simulink model "test_stepper"  (R2020b)
settings: Solver=VariableStepAuto  StartTime=0.0  StopTime=10.0  RelTol=1e-3
undefined symbols (not defined in the file): stepper
settings Model: Creator=Utente  LastModifiedBy=Utente
settings SolverCC: ZeroCrossAlgorithm=Adaptive
settings DebuggingCC: IgnoredZcDiagnostic=none

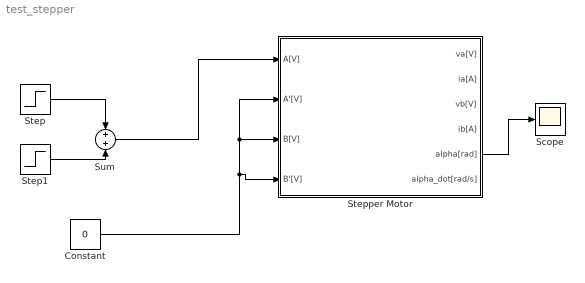
== system test_stepper ==
  Constant : Constant  Value=0
  Scope : Scope
  Step : Step  Time=0  After=9  SampleTime=0
  Step1 : Step  Time=0.0001  After=-1  SampleTime=0
  Stepper Motor : Subsystem
  Sum : Sum
  wires:
  Step/1 -> Sum/1
  Step1/1 -> Sum/2
  Sum/1 -> Stepper Motor/1(A[V])
  Constant/1 -> Stepper Motor/4(B'[V]), Stepper Motor/3(B[V]), Stepper Motor/2(A'[V])
  Stepper Motor/5(alpha[rad]) -> Scope/1

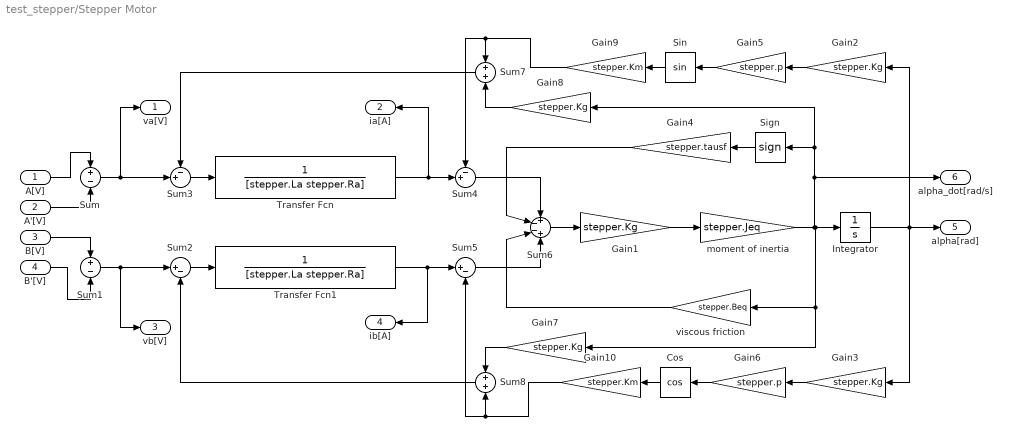
== system test_stepper/Stepper Motor ==
  A[V] : Inport
  A'[V] : Inport  Port=2
  B[V] : Inport  Port=3
  B'[V] : Inport  Port=4
  Cos : Trigonometry  Operator=cos
  Gain{1..3,7..8} (5 alike) : Gain  Gain=stepper.Kg
  Gain10 : Gain  Gain=stepper.Km
  Gain4 : Gain  Gain=stepper.tausf
  Gain5 : Gain  Gain=stepper.p
  Gain6 : Gain  Gain=stepper.p
  Gain9 : Gain  Gain=stepper.Km
  Integrator : Integrator
  Sign : Signum  ZeroCross=off
  Sin : Trigonometry
  Sum : Sum  Inputs=+|-
  Sum1 : Sum  Inputs=+|-
  Sum2 : Sum  Inputs=|+-
  Sum3 : Sum  Inputs=-+|
  Sum4 : Sum  Inputs=-+|
  Sum5 : Sum  Inputs=|+-
  Sum6 : Sum  Inputs=+--+
  Sum7 : Sum
  Sum8 : Sum
  Transfer Fcn : TransferFcn  Denominator=[stepper.La stepper.Ra]
  Transfer Fcn1 : TransferFcn  Denominator=[stepper.La stepper.Ra]
  moment of inertia : Gain  Gain=stepper.Jeq
  viscous friction : Gain  Gain=stepper.Beq
  va[V] : Outport
  ia[A] : Outport  Port=2
  vb[V] : Outport  Port=3
  ib[A] : Outport  Port=4
  alpha[rad] : Outport  Port=5
  alpha_dot[rad/s] : Outport  Port=6
  wires:
  A'[V]/1 -> Sum/2
  A[V]/1 -> Sum/1
  Sum/1 -> Sum3/2, va[V]/1
  B[V]/1 -> Sum1/1
  B'[V]/1 -> Sum1/2
  Sum1/1 -> Sum2/1, vb[V]/1
  Integrator/1 -> Gain3/1, Gain2/1, alpha[rad]/1
  Sum3/1 -> Transfer Fcn/1
  Sum2/1 -> Transfer Fcn1/1
  Sum4/1 -> Sum6/1
  Sum5/1 -> Sum6/4
  Sum6/1 -> Gain1/1
  Gain1/1 -> moment of inertia/1
  moment of inertia/1 -> viscous friction/1, Gain7/1, Integrator/1, Sign/1, Gain8/1, alpha_dot[rad/s]/1
  viscous friction/1 -> Sum6/3
  Gain4/1 -> Sum6/2
  Transfer Fcn/1 -> ia[A]/1, Sum4/2
  Transfer Fcn1/1 -> ib[A]/1, Sum5/1
  Gain2/1 -> Gain5/1
  Gain5/1 -> Sin/1
  Gain6/1 -> Cos/1
  Gain3/1 -> Gain6/1
  Gain8/1 -> Sum7/2
  Sin/1 -> Gain9/1
  Gain7/1 -> Sum8/1
  Cos/1 -> Gain10/1
  Sum8/1 -> Sum2/2
  Sum7/1 -> Sum3/1
  Gain9/1 -> Sum4/1, Sum7/1
  Gain10/1 -> Sum8/2, Sum5/2
  Sign/1 -> Gain4/1
